simulink model "dft_polyphase_channelizer_32_by_8"  (R2018b)
settings: Solver=FixedStepDiscrete  StartTime=0.0  StopTime=t(end)  RelTol=1e-3  EnableMultiTasking=on
InitFcn:
  | M = 32; % Number of channels in the filter bank.
  | N = 8;  % Number of taps in each FIR filter.
  | n_out = 4000; % Number of output samples
  | datatypeselector = 'hdl'; % 'double' 'single' 'hdl' 'dsp'
  | fidatatype = 'Fixed'; % 'Fixed' 'ScaledDouble'
  | [T,B,U,b,u,t,fs] = generate_inputs(M,N,n_out,datatypeselector,fidatatype);
values from neighbouring files (symbols this model uses):
  B = cast(B,'like',T.fir_filter.coeff)    [generate_inputs.m]    (also in test_real_resource_shared_QR.m = cast(B,'like',A))
  fs = n    [generate_inputs.m]
  T = dft_polyphase_filter_types(datatypeselector,fidatatype,prototypevalue,max(abs(b)))    [generate_inputs.m]
(part 1 of 2)
settings Model: FPTRunName=ScaledDouble  Creator=tbryan  LastModifiedBy=tbryan
settings SolverCC: AutoInsertRateTranBlk=on
settings OptimizationCC: LifeSpan=inf
settings DebuggingCC: ParameterDowncastMsg=none  ParameterOverflowMsg=none  ParameterPrecisionLossMsg=none  ParameterTunabilityLossMsg=none  AllowSymbolicDim=off  LibraryContextMissingDiagnostic=none  SFUnexpectedBacktrackingDiag=warning  SFNoUnconditionalDefaultTransitionDiag=warning  SFExecutionAtInitializationDiag=none
settings HardwareCC: ProdBitPerPointer=32  ProdBitPerSizeT=32  ProdBitPerPtrDiffT=32  ProdLargestAtomicFloat=None  ProdIntDivRoundTo=Undefined  ProdEndianess=Unspecified  ProdWordSize=32  ProdHWDeviceType=ASIC/FPGA->ASIC/FPGA  TargetBitPerLong=64  TargetBitPerPointer=64  TargetBitPerSizeT=64  TargetBitPerPtrDiffT=64  TargetLongLongMode=on  TargetIntDivRoundTo=Zero  TargetEndianess=LittleEndian  TargetWordSize=64  TargetHWDeviceType=MATLAB Host  ProdEqTarget=off
settings SFSimCC: SimUseLocalCustomCode=off
settings RTWCC: RTWUseLocalCustomCode=off
settings CodeAppCC: StateflowObjectComments=on
settings GRTTargetCC: TargetLangStandard=C89/C90 (ANSI)  GeneratePreprocessorConditionals=Disable all
settings ConfigComp: CovMetricSettings=dw  CovHtmlReporting=on  CovSaveCumulativeToWorkspaceVar=on  CovSaveSingleToWorkspaceVar=on  CovExternalEMLEnable=off

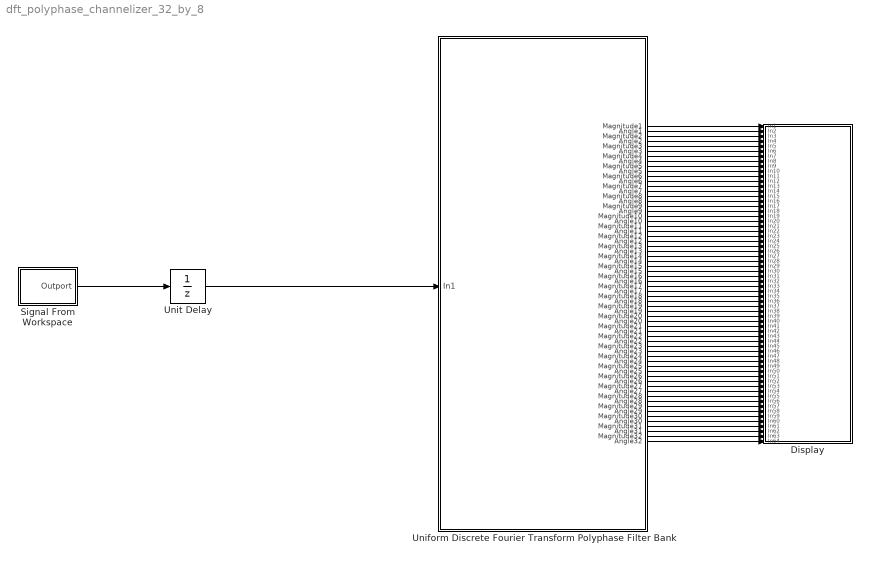
== system dft_polyphase_channelizer_32_by_8 ==
  Display : Subsystem
  Signal From Workspace : Subsystem  mask(Signal From Workspace){X=u, Ts=1/fs, nsamps=1, OutputAfterFinalValue=Setting to zero, ignoreOrWarnInputAndFrameLengths=off, OutputFrames=off}
      mask prompts: X "Signal:"; Ts "Sample time:"; nsamps "Samples per frame:"; OutputAfterFinalValue "Form output after final data value by:"; ignoreOrWarnInputAndFrameLengths "Warn when frame size does not evenly divide input length"; OutputFrames "Output Frames"
      mask help:
      | Output signal samples obtained from the MATLAB workspace at successive sample times.  A signal matrix is interpreted as having one channel per column.  Signal columns may be buffered into frames by specifying a number of samples per frame greater than 1.
      |
      | An M x N x P signal array outputs M x N matrices at successive sample times.  The samples per frame must be equal to 1 for three-dimensional signal arrays.
      mask init:
      | dispX = get_param(gcbh, 'X');
      | [s,Ts] = dspblksfw2('init', X,Ts,nsamps);
      mask Help: eval('blocksethelp');
      mask TypeOptions OutputAfterFinalValue: Setting to zero | Holding final value | Cyclic repetition
      mask Callback OutputAfterFinalValue: dspblksfw2
      mask Display: disp(dispX)
  Uniform Discrete Fourier Transform Polyphase Filter Bank : Subsystem
  Unit Delay : UnitDelay  SampleTime=1/fs
  wires:
  Unit Delay/1 -> Uniform Discrete Fourier Transform Polyphase Filter Bank/1(In1)
  Signal From Workspace/1(Outport) -> Unit Delay/1
  Uniform Discrete Fourier Transform Polyphase Filter Bank/1(Magnitude1) -> Display/1(In1)
  Uniform Discrete Fourier Transform Polyphase Filter Bank/2(Angle1) -> Display/2(In2)
  Uniform Discrete Fourier Transform Polyphase Filter Bank/3(Magnitude2) -> Display/3(In3)
  Uniform Discrete Fourier Transform Polyphase Filter Bank/4(Angle2) -> Display/4(In4)
  Uniform Discrete Fourier Transform Polyphase Filter Bank/5(Magnitude3) -> Display/5(In5)
  Uniform Discrete Fourier Transform Polyphase Filter Bank/6(Angle3) -> Display/6(In6)
  Uniform Discrete Fourier Transform Polyphase Filter Bank/7(Magnitude4) -> Display/7(In7)
  Uniform Discrete Fourier Transform Polyphase Filter Bank/8(Angle4) -> Display/8(In8)
  Uniform Discrete Fourier Transform Polyphase Filter Bank/9(Magnitude5) -> Display/9(In9)
  Uniform Discrete Fourier Transform Polyphase Filter Bank/10(Angle5) -> Display/10(In10)
  Uniform Discrete Fourier Transform Polyphase Filter Bank/11(Magnitude6) -> Display/11(In11)
  Uniform Discrete Fourier Transform Polyphase Filter Bank/12(Angle6) -> Display/12(In12)
  Uniform Discrete Fourier Transform Polyphase Filter Bank/13(Magnitude7) -> Display/13(In13)
  Uniform Discrete Fourier Transform Polyphase Filter Bank/14(Angle7) -> Display/14(In14)
  Uniform Discrete Fourier Transform Polyphase Filter Bank/15(Magnitude8) -> Display/15(In15)
  Uniform Discrete Fourier Transform Polyphase Filter Bank/16(Angle8) -> Display/16(In16)
  Uniform Discrete Fourier Transform Polyphase Filter Bank/17(Magnitude9) -> Display/17(In17)
  Uniform Discrete Fourier Transform Polyphase Filter Bank/18(Angle9) -> Display/18(In18)
  Uniform Discrete Fourier Transform Polyphase Filter Bank/19(Magnitude10) -> Display/19(In19)
  Uniform Discrete Fourier Transform Polyphase Filter Bank/20(Angle10) -> Display/20(In20)
  Uniform Discrete Fourier Transform Polyphase Filter Bank/21(Magnitude11) -> Display/21(In21)
  Uniform Discrete Fourier Transform Polyphase Filter Bank/22(Angle11) -> Display/22(In22)
  Uniform Discrete Fourier Transform Polyphase Filter Bank/23(Magnitude12) -> Display/23(In23)
  Uniform Discrete Fourier Transform Polyphase Filter Bank/24(Angle12) -> Display/24(In24)
  Uniform Discrete Fourier Transform Polyphase Filter Bank/25(Magnitude13) -> Display/25(In25)
  Uniform Discrete Fourier Transform Polyphase Filter Bank/26(Angle13) -> Display/26(In26)
  Uniform Discrete Fourier Transform Polyphase Filter Bank/27(Magnitude14) -> Display/27(In27)
  Uniform Discrete Fourier Transform Polyphase Filter Bank/28(Angle14) -> Display/28(In28)
  Uniform Discrete Fourier Transform Polyphase Filter Bank/29(Magnitude15) -> Display/29(In29)
  Uniform Discrete Fourier Transform Polyphase Filter Bank/30(Angle15) -> Display/30(In30)
  Uniform Discrete Fourier Transform Polyphase Filter Bank/31(Magnitude16) -> Display/31(In31)
  Uniform Discrete Fourier Transform Polyphase Filter Bank/32(Angle16) -> Display/32(In32)
  Uniform Discrete Fourier Transform Polyphase Filter Bank/33(Magnitude17) -> Display/33(In33)
  Uniform Discrete Fourier Transform Polyphase Filter Bank/34(Angle17) -> Display/34(In34)
  Uniform Discrete Fourier Transform Polyphase Filter Bank/35(Magnitude18) -> Display/35(In35)
  Uniform Discrete Fourier Transform Polyphase Filter Bank/36(Angle18) -> Display/36(In36)
  Uniform Discrete Fourier Transform Polyphase Filter Bank/37(Magnitude19) -> Display/37(In37)
  Uniform Discrete Fourier Transform Polyphase Filter Bank/38(Angle19) -> Display/38(In38)
  Uniform Discrete Fourier Transform Polyphase Filter Bank/39(Magnitude20) -> Display/39(In39)
  Uniform Discrete Fourier Transform Polyphase Filter Bank/40(Angle20) -> Display/40(In40)
  Uniform Discrete Fourier Transform Polyphase Filter Bank/41(Magnitude21) -> Display/41(In41)
  Uniform Discrete Fourier Transform Polyphase Filter Bank/42(Angle21) -> Display/42(In42)
  Uniform Discrete Fourier Transform Polyphase Filter Bank/43(Magnitude22) -> Display/43(In43)
  Uniform Discrete Fourier Transform Polyphase Filter Bank/44(Angle22) -> Display/44(In44)
  Uniform Discrete Fourier Transform Polyphase Filter Bank/45(Magnitude23) -> Display/45(In45)
  Uniform Discrete Fourier Transform Polyphase Filter Bank/46(Angle23) -> Display/46(In46)
  Uniform Discrete Fourier Transform Polyphase Filter Bank/47(Magnitude24) -> Display/47(In47)
  Uniform Discrete Fourier Transform Polyphase Filter Bank/48(Angle24) -> Display/48(In48)
  Uniform Discrete Fourier Transform Polyphase Filter Bank/49(Magnitude25) -> Display/49(In49)
  Uniform Discrete Fourier Transform Polyphase Filter Bank/50(Angle25) -> Display/50(In50)
  Uniform Discrete Fourier Transform Polyphase Filter Bank/51(Magnitude26) -> Display/51(In51)
  Uniform Discrete Fourier Transform Polyphase Filter Bank/52(Angle26) -> Display/52(In52)
  Uniform Discrete Fourier Transform Polyphase Filter Bank/53(Magnitude27) -> Display/53(In53)
  Uniform Discrete Fourier Transform Polyphase Filter Bank/54(Angle27) -> Display/54(In54)
  Uniform Discrete Fourier Transform Polyphase Filter Bank/55(Magnitude28) -> Display/55(In55)
  Uniform Discrete Fourier Transform Polyphase Filter Bank/56(Angle28) -> Display/56(In56)
  Uniform Discrete Fourier Transform Polyphase Filter Bank/57(Magnitude29) -> Display/57(In57)
  Uniform Discrete Fourier Transform Polyphase Filter Bank/58(Angle29) -> Display/58(In58)
  Uniform Discrete Fourier Transform Polyphase Filter Bank/59(Magnitude30) -> Display/59(In59)
  Uniform Discrete Fourier Transform Polyphase Filter Bank/60(Angle30) -> Display/60(In60)
  Uniform Discrete Fourier Transform Polyphase Filter Bank/61(Magnitude31) -> Display/61(In61)
  Uniform Discrete Fourier Transform Polyphase Filter Bank/62(Angle31) -> Display/62(In62)
  Uniform Discrete Fourier Transform Polyphase Filter Bank/63(Magnitude32) -> Display/63(In63)
  Uniform Discrete Fourier Transform Polyphase Filter Bank/64(Angle32) -> Display/64(In64)

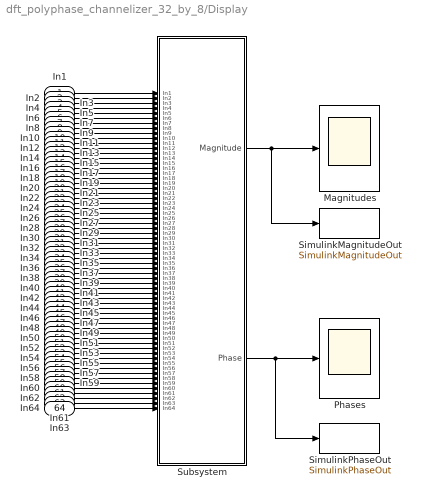
== system dft_polyphase_channelizer_32_by_8/Display ==
  In1 : Inport
  In2 : Inport  Port=2
  In3 : Inport  Port=3
  In4 : Inport  Port=4
  In5 : Inport  Port=5
  In6 : Inport  Port=6
  In7 : Inport  Port=7
  In8 : Inport  Port=8
  In9 : Inport  Port=9
  In10 : Inport  Port=10
  In11 : Inport  Port=11
  In12 : Inport  Port=12
  In13 : Inport  Port=13
  In14 : Inport  Port=14
  In15 : Inport  Port=15
  In16 : Inport  Port=16
  In17 : Inport  Port=17
  In18 : Inport  Port=18
  In19 : Inport  Port=19
  In20 : Inport  Port=20
  In21 : Inport  Port=21
  In22 : Inport  Port=22
  In23 : Inport  Port=23
  In24 : Inport  Port=24
  In25 : Inport  Port=25
  In26 : Inport  Port=26
  In27 : Inport  Port=27
  In28 : Inport  Port=28
  In29 : Inport  Port=29
  In30 : Inport  Port=30
  In31 : Inport  Port=31
  In32 : Inport  Port=32
  In33 : Inport  Port=33
  In34 : Inport  Port=34
  In35 : Inport  Port=35
  In36 : Inport  Port=36
  In37 : Inport  Port=37
  In38 : Inport  Port=38
  In39 : Inport  Port=39
  In40 : Inport  Port=40
  In41 : Inport  Port=41
  In42 : Inport  Port=42
  In43 : Inport  Port=43
  In44 : Inport  Port=44
  In45 : Inport  Port=45
  In46 : Inport  Port=46
  In47 : Inport  Port=47
  In48 : Inport  Port=48
  In49 : Inport  Port=49
  In50 : Inport  Port=50
  In51 : Inport  Port=51
  In52 : Inport  Port=52
  In53 : Inport  Port=53
  In54 : Inport  Port=54
  In55 : Inport  Port=55
  In56 : Inport  Port=56
  In57 : Inport  Port=57
  In58 : Inport  Port=58
  In59 : Inport  Port=59
  In60 : Inport  Port=60
  In61 : Inport  Port=61
  In62 : Inport  Port=62
  In63 : Inport  Port=63
  In64 : Inport  Port=64
  Magnitudes : Scope
  Phases : Scope
  SimulinkMagnitudeOut : ToWorkspace  VariableName=SimulinkMagnitudeOut  SampleTime=-1
      settings: Save2DSignal=2-D array (concatenate along first dimension)
  SimulinkPhaseOut : ToWorkspace  VariableName=SimulinkPhaseOut  SampleTime=-1
      settings: Save2DSignal=2-D array (concatenate along first dimension)
  Subsystem : Subsystem
  wires:
  In8/1 -> Subsystem/8(In8)
  In43/1 -> Subsystem/43(In43)
  In21/1 -> Subsystem/21(In21)
  In35/1 -> Subsystem/35(In35)
  In33/1 -> Subsystem/33(In33)
  In26/1 -> Subsystem/26(In26)
  In30/1 -> Subsystem/30(In30)
  In27/1 -> Subsystem/27(In27)
  In23/1 -> Subsystem/23(In23)
  In20/1 -> Subsystem/20(In20)
  In5/1 -> Subsystem/5(In5)
  In63/1 -> Subsystem/63(In63)
  In10/1 -> Subsystem/10(In10)
  In61/1 -> Subsystem/61(In61)
  In41/1 -> Subsystem/41(In41)
  In6/1 -> Subsystem/6(In6)
  In49/1 -> Subsystem/49(In49)
  In53/1 -> Subsystem/53(In53)
  In47/1 -> Subsystem/47(In47)
  In55/1 -> Subsystem/55(In55)
  In13/1 -> Subsystem/13(In13)
  In32/1 -> Subsystem/32(In32)
  In14/1 -> Subsystem/14(In14)
  In38/1 -> Subsystem/38(In38)
  In17/1 -> Subsystem/17(In17)
  In1/1 -> Subsystem/1(In1)
  In62/1 -> Subsystem/62(In62)
  In46/1 -> Subsystem/46(In46)
  In44/1 -> Subsystem/44(In44)
  In58/1 -> Subsystem/58(In58)
  In12/1 -> Subsystem/12(In12)
  In19/1 -> Subsystem/19(In19)
  In15/1 -> Subsystem/15(In15)
  In16/1 -> Subsystem/16(In16)
  In18/1 -> Subsystem/18(In18)
  In24/1 -> Subsystem/24(In24)
  In29/1 -> Subsystem/29(In29)
  In2/1 -> Subsystem/2(In2)
  In3/1 -> Subsystem/3(In3)
  In7/1 -> Subsystem/7(In7)
  In4/1 -> Subsystem/4(In4)
  In28/1 -> Subsystem/28(In28)
  In9/1 -> Subsystem/9(In9)
  In22/1 -> Subsystem/22(In22)
  Subsystem/2(Phase) -> SimulinkPhaseOut/1, Phases/1
  In57/1 -> Subsystem/57(In57)
  In36/1 -> Subsystem/36(In36)
  In50/1 -> Subsystem/50(In50)
  In34/1 -> Subsystem/34(In34)
  In56/1 -> Subsystem/56(In56)
  In11/1 -> Subsystem/11(In11)
  In64/1 -> Subsystem/64(In64)
  Subsystem/1(Magnitude) -> SimulinkMagnitudeOut/1, Magnitudes/1
  In25/1 -> Subsystem/25(In25)
  In59/1 -> Subsystem/59(In59)
  In39/1 -> Subsystem/39(In39)
  In45/1 -> Subsystem/45(In45)
  In42/1 -> Subsystem/42(In42)
  In52/1 -> Subsystem/52(In52)
  In60/1 -> Subsystem/60(In60)
  In48/1 -> Subsystem/48(In48)
  In51/1 -> Subsystem/51(In51)
  In54/1 -> Subsystem/54(In54)
  In31/1 -> Subsystem/31(In31)
  In37/1 -> Subsystem/37(In37)
  In40/1 -> Subsystem/40(In40)

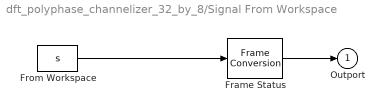
== system dft_polyphase_channelizer_32_by_8/Signal From Workspace ==
  Frame Status : FrameConversion  OutFrame=Sample-based
  From Workspace : FromWorkspace  VariableName=s  SampleTime=Ts  Interpolate=off  OutputAfterFinalValue=Setting to zero
  Outport : Outport  InitialOutput=0
  wires:
  Frame Status/1 -> Outport/1
  From Workspace/1 -> Frame Status/1

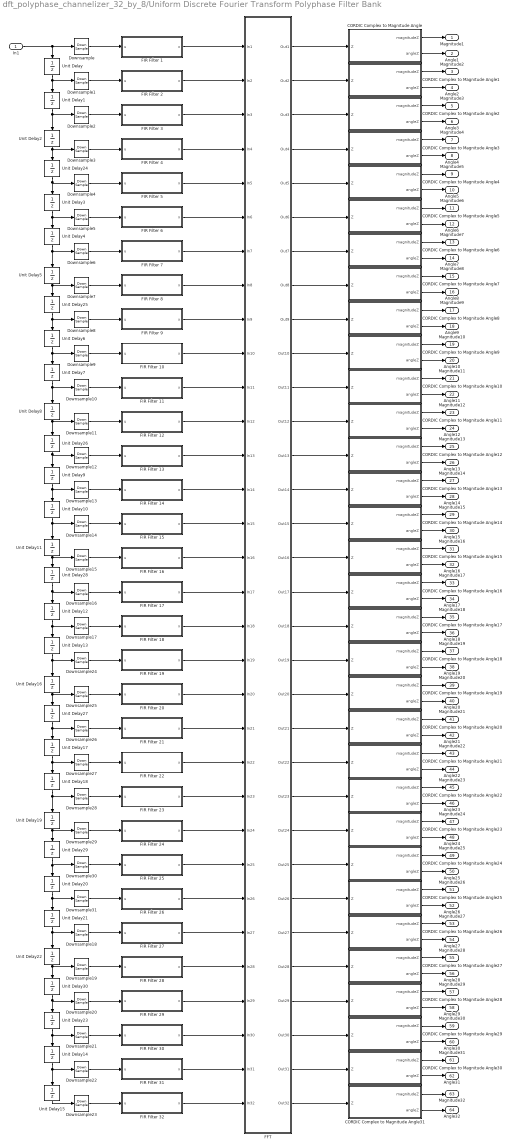
== system dft_polyphase_channelizer_32_by_8/Uniform Discrete Fourier Transform Polyphase Filter Bank ==
  In1 : Inport
  " CORDIC Complex to Magnitude Angle" : MATLAB Function  TreatAsAtomicUnit=on
  " CORDIC Complex to Magnitude Angle1" : MATLAB Function  TreatAsAtomicUnit=on
  " CORDIC Complex to Magnitude Angle10" : MATLAB Function  TreatAsAtomicUnit=on
  " CORDIC Complex to Magnitude Angle11" : MATLAB Function  TreatAsAtomicUnit=on
  " CORDIC Complex to Magnitude Angle12" : MATLAB Function  TreatAsAtomicUnit=on
  " CORDIC Complex to Magnitude Angle13" : MATLAB Function  TreatAsAtomicUnit=on
  " CORDIC Complex to Magnitude Angle14" : MATLAB Function  TreatAsAtomicUnit=on
  " CORDIC Complex to Magnitude Angle15" : MATLAB Function  TreatAsAtomicUnit=on
  " CORDIC Complex to Magnitude Angle16" : MATLAB Function  TreatAsAtomicUnit=on
  " CORDIC Complex to Magnitude Angle17" : MATLAB Function  TreatAsAtomicUnit=on
  " CORDIC Complex to Magnitude Angle18" : MATLAB Function  TreatAsAtomicUnit=on
  " CORDIC Complex to Magnitude Angle19" : MATLAB Function  TreatAsAtomicUnit=on
  " CORDIC Complex to Magnitude Angle2" : MATLAB Function  TreatAsAtomicUnit=on
  " CORDIC Complex to Magnitude Angle20" : MATLAB Function  TreatAsAtomicUnit=on
  " CORDIC Complex to Magnitude Angle21" : MATLAB Function  TreatAsAtomicUnit=on
  " CORDIC Complex to Magnitude Angle22" : MATLAB Function  TreatAsAtomicUnit=on
  " CORDIC Complex to Magnitude Angle23" : MATLAB Function  TreatAsAtomicUnit=on
  " CORDIC Complex to Magnitude Angle24" : MATLAB Function  TreatAsAtomicUnit=on
  " CORDIC Complex to Magnitude Angle25" : MATLAB Function  TreatAsAtomicUnit=on
  " CORDIC Complex to Magnitude Angle26" : MATLAB Function  TreatAsAtomicUnit=on
  " CORDIC Complex to Magnitude Angle27" : MATLAB Function  TreatAsAtomicUnit=on
  " CORDIC Complex to Magnitude Angle28" : MATLAB Function  TreatAsAtomicUnit=on
  " CORDIC Complex to Magnitude Angle29" : MATLAB Function  TreatAsAtomicUnit=on
  " CORDIC Complex to Magnitude Angle3" : MATLAB Function  TreatAsAtomicUnit=on
  " CORDIC Complex to Magnitude Angle30" : MATLAB Function  TreatAsAtomicUnit=on
  " CORDIC Complex to Magnitude Angle31" : MATLAB Function  TreatAsAtomicUnit=on
  " CORDIC Complex to Magnitude Angle4" : MATLAB Function  TreatAsAtomicUnit=on
  " CORDIC Complex to Magnitude Angle5" : MATLAB Function  TreatAsAtomicUnit=on
  " CORDIC Complex to Magnitude Angle6" : MATLAB Function  TreatAsAtomicUnit=on
  " CORDIC Complex to Magnitude Angle7" : MATLAB Function  TreatAsAtomicUnit=on
  " CORDIC Complex to Magnitude Angle8" : MATLAB Function  TreatAsAtomicUnit=on
  " CORDIC Complex to Magnitude Angle9" : MATLAB Function  TreatAsAtomicUnit=on
  Downsample{,1..31} (32 alike) : DownSample  N=M  RateOptions=Allow multirate processing
  FFT : Subsystem
      mask Display: disp('FFT')
  FIR Filter 1 : MATLAB Function  TreatAsAtomicUnit=on  mask{b=B(1,:), T=T.fir_filter}
      mask prompts: b "Coefficients: b from MATLAB's filter(b,1,x)"
  FIR Filter 10 : MATLAB Function  TreatAsAtomicUnit=on  mask{b=B(10,:), T=T.fir_filter}
      mask prompts: b "Coefficients: b from MATLAB's filter(b,1,x)"
  FIR Filter 11 : MATLAB Function  TreatAsAtomicUnit=on  mask{b=B(11,:), T=T.fir_filter}
      mask prompts: b "Coefficients: b from MATLAB's filter(b,1,x)"
  FIR Filter 12 : MATLAB Function  TreatAsAtomicUnit=on  mask{b=B(12,:), T=T.fir_filter}
      mask prompts: b "Coefficients: b from MATLAB's filter(b,1,x)"
  FIR Filter 13 : MATLAB Function  TreatAsAtomicUnit=on  mask{b=B(13,:), T=T.fir_filter}
      mask prompts: b "Coefficients: b from MATLAB's filter(b,1,x)"
  FIR Filter 14 : MATLAB Function  TreatAsAtomicUnit=on  mask{b=B(14,:), T=T.fir_filter}
      mask prompts: b "Coefficients: b from MATLAB's filter(b,1,x)"
  FIR Filter 15 : MATLAB Function  TreatAsAtomicUnit=on  mask{b=B(15,:), T=T.fir_filter}
      mask prompts: b "Coefficients: b from MATLAB's filter(b,1,x)"
  FIR Filter 16 : MATLAB Function  TreatAsAtomicUnit=on  mask{b=B(16,:), T=T.fir_filter}
      mask prompts: b "Coefficients: b from MATLAB's filter(b,1,x)"
  FIR Filter 17 : MATLAB Function  TreatAsAtomicUnit=on  mask{b=B(17,:), T=T.fir_filter}
      mask prompts: b "Coefficients: b from MATLAB's filter(b,1,x)"
  FIR Filter 18 : MATLAB Function  TreatAsAtomicUnit=on  mask{b=B(18,:), T=T.fir_filter}
      mask prompts: b "Coefficients: b from MATLAB's filter(b,1,x)"
  FIR Filter 19 : MATLAB Function  TreatAsAtomicUnit=on  mask{b=B(19,:), T=T.fir_filter}
      mask prompts: b "Coefficients: b from MATLAB's filter(b,1,x)"
  FIR Filter 2 : MATLAB Function  TreatAsAtomicUnit=on  mask{b=B(2,:), T=T.fir_filter}
      mask prompts: b "Coefficients: b from MATLAB's filter(b,1,x)"
  FIR Filter 20 : MATLAB Function  TreatAsAtomicUnit=on  mask{b=B(20,:), T=T.fir_filter}
      mask prompts: b "Coefficients: b from MATLAB's filter(b,1,x)"
  FIR Filter 21 : MATLAB Function  TreatAsAtomicUnit=on  mask{b=B(21,:), T=T.fir_filter}
      mask prompts: b "Coefficients: b from MATLAB's filter(b,1,x)"
  FIR Filter 22 : MATLAB Function  TreatAsAtomicUnit=on  mask{b=B(22,:), T=T.fir_filter}
      mask prompts: b "Coefficients: b from MATLAB's filter(b,1,x)"
  FIR Filter 23 : MATLAB Function  TreatAsAtomicUnit=on  mask{b=B(23,:), T=T.fir_filter}
      mask prompts: b "Coefficients: b from MATLAB's filter(b,1,x)"
  FIR Filter 24 : MATLAB Function  TreatAsAtomicUnit=on  mask{b=B(24,:), T=T.fir_filter}
      mask prompts: b "Coefficients: b from MATLAB's filter(b,1,x)"
  FIR Filter 25 : MATLAB Function  TreatAsAtomicUnit=on  mask{b=B(25,:), T=T.fir_filter}
      mask prompts: b "Coefficients: b from MATLAB's filter(b,1,x)"
  FIR Filter 26 : MATLAB Function  TreatAsAtomicUnit=on  mask{b=B(26,:), T=T.fir_filter}
      mask prompts: b "Coefficients: b from MATLAB's filter(b,1,x)"
  FIR Filter 27 : MATLAB Function  TreatAsAtomicUnit=on  mask{b=B(27,:), T=T.fir_filter}
      mask prompts: b "Coefficients: b from MATLAB's filter(b,1,x)"
  FIR Filter 28 : MATLAB Function  TreatAsAtomicUnit=on  mask{b=B(28,:), T=T.fir_filter}
      mask prompts: b "Coefficients: b from MATLAB's filter(b,1,x)"
  FIR Filter 29 : MATLAB Function  TreatAsAtomicUnit=on  mask{b=B(29,:), T=T.fir_filter}
      mask prompts: b "Coefficients: b from MATLAB's filter(b,1,x)"
  FIR Filter 3 : MATLAB Function  TreatAsAtomicUnit=on  mask{b=B(3,:), T=T.fir_filter}
      mask prompts: b "Coefficients: b from MATLAB's filter(b,1,x)"
  FIR Filter 30 : MATLAB Function  TreatAsAtomicUnit=on  mask{b=B(30,:), T=T.fir_filter}
      mask prompts: b "Coefficients: b from MATLAB's filter(b,1,x)"
  FIR Filter 31 : MATLAB Function  TreatAsAtomicUnit=on  mask{b=B(31,:), T=T.fir_filter}
      mask prompts: b "Coefficients: b from MATLAB's filter(b,1,x)"
  FIR Filter 32 : MATLAB Function  TreatAsAtomicUnit=on  mask{b=B(32,:), T=T.fir_filter}
      mask prompts: b "Coefficients: b from MATLAB's filter(b,1,x)"
  FIR Filter 4 : MATLAB Function  TreatAsAtomicUnit=on  mask{b=B(4,:), T=T.fir_filter}
      mask prompts: b "Coefficients: b from MATLAB's filter(b,1,x)"
  FIR Filter 5 : MATLAB Function  TreatAsAtomicUnit=on  mask{b=B(5,:), T=T.fir_filter}
      mask prompts: b "Coefficients: b from MATLAB's filter(b,1,x)"
  FIR Filter 6 : MATLAB Function  TreatAsAtomicUnit=on  mask{b=B(6,:), T=T.fir_filter}
      mask prompts: b "Coefficients: b from MATLAB's filter(b,1,x)"
  FIR Filter 7 : MATLAB Function  TreatAsAtomicUnit=on  mask{b=B(7,:), T=T.fir_filter}
      mask prompts: b "Coefficients: b from MATLAB's filter(b,1,x)"
  FIR Filter 8 : MATLAB Function  TreatAsAtomicUnit=on  mask{b=B(8,:), T=T.fir_filter}
      mask prompts: b "Coefficients: b from MATLAB's filter(b,1,x)"
  FIR Filter 9 : MATLAB Function  TreatAsAtomicUnit=on  mask{b=B(9,:), T=T.fir_filter}
      mask prompts: b "Coefficients: b from MATLAB's filter(b,1,x)"
  Unit Delay{,1..30} (31 alike) : UnitDelay  SampleTime=-1
  Magnitude1 : Outport
  Angle1 : Outport  Port=2
  Magnitude2 : Outport  Port=3
  Angle2 : Outport  Port=4
  Magnitude3 : Outport  Port=5
  Angle3 : Outport  Port=6
  Magnitude4 : Outport  Port=7
  Angle4 : Outport  Port=8
  Magnitude5 : Outport  Port=9
  Angle5 : Outport  Port=10
  Magnitude6 : Outport  Port=11
  Angle6 : Outport  Port=12
  Magnitude7 : Outport  Port=13
  Angle7 : Outport  Port=14
  Magnitude8 : Outport  Port=15
  Angle8 : Outport  Port=16
  Magnitude9 : Outport  Port=17
  Angle9 : Outport  Port=18
  Magnitude10 : Outport  Port=19
  Angle10 : Outport  Port=20
  Magnitude11 : Outport  Port=21
  Angle11 : Outport  Port=22
  Magnitude12 : Outport  Port=23
  Angle12 : Outport  Port=24
  Magnitude13 : Outport  Port=25
  Angle13 : Outport  Port=26
  Magnitude14 : Outport  Port=27
  Angle14 : Outport  Port=28
  Magnitude15 : Outport  Port=29
  Angle15 : Outport  Port=30
  Magnitude16 : Outport  Port=31
  Angle16 : Outport  Port=32
  Magnitude17 : Outport  Port=33
  Angle17 : Outport  Port=34
  Magnitude18 : Outport  Port=35
  Angle18 : Outport  Port=36
  Magnitude19 : Outport  Port=37
  Angle19 : Outport  Port=38
  Magnitude20 : Outport  Port=39
  Angle20 : Outport  Port=40
  Magnitude21 : Outport  Port=41
  Angle21 : Outport  Port=42
  Magnitude22 : Outport  Port=43
  Angle22 : Outport  Port=44
  Magnitude23 : Outport  Port=45
  Angle23 : Outport  Port=46
  Magnitude24 : Outport  Port=47
  Angle24 : Outport  Port=48
  Magnitude25 : Outport  Port=49
  Angle25 : Outport  Port=50
  Magnitude26 : Outport  Port=51
  Angle26 : Outport  Port=52
  Magnitude27 : Outport  Port=53
  Angle27 : Outport  Port=54
  Magnitude28 : Outport  Port=55
  Angle28 : Outport  Port=56
  Magnitude29 : Outport  Port=57
  Angle29 : Outport  Port=58
  Magnitude30 : Outport  Port=59
  Angle30 : Outport  Port=60
  Magnitude31 : Outport  Port=61
  Angle31 : Outport  Port=62
  Magnitude32 : Outport  Port=63
  Angle32 : Outport  Port=64
  wires:
  " CORDIC Complex to Magnitude Angle1"/2(angleZ) -> Angle2/1
  " CORDIC Complex to Magnitude Angle"/1(magnitudeZ) -> Magnitude1/1
  " CORDIC Complex to Magnitude Angle2"/2(angleZ) -> Angle3/1
  " CORDIC Complex to Magnitude Angle3"/2(angleZ) -> Angle4/1
  " CORDIC Complex to Magnitude Angle2"/1(magnitudeZ) -> Magnitude3/1
  " CORDIC Complex to Magnitude Angle"/2(angleZ) -> Angle1/1
  " CORDIC Complex to Magnitude Angle3"/1(magnitudeZ) -> Magnitude4/1
  Downsample/1 -> FIR Filter 1/1(u)
  Unit Delay/1 -> Unit Delay1/1, Downsample1/1
  Unit Delay1/1 -> Unit Delay2/1, Downsample2/1
  Unit Delay2/1 -> Unit Delay24/1, Downsample3/1
  " CORDIC Complex to Magnitude Angle1"/1(magnitudeZ) -> Magnitude2/1
  Unit Delay3/1 -> Unit Delay4/1, Downsample5/1
  Unit Delay4/1 -> Unit Delay5/1, Downsample6/1
  Unit Delay6/1 -> Unit Delay7/1, Downsample9/1
  Unit Delay7/1 -> Unit Delay8/1, Downsample10/1
  Unit Delay8/1 -> Unit Delay26/1, Downsample11/1
  Unit Delay9/1 -> Unit Delay10/1, Downsample13/1
  Unit Delay10/1 -> Unit Delay11/1, Downsample14/1
  Unit Delay11/1 -> Unit Delay28/1, Downsample15/1
  Unit Delay12/1 -> Unit Delay13/1, Downsample17/1
  Unit Delay13/1 -> Unit Delay16/1, Downsample24/1
  Unit Delay16/1 -> Unit Delay27/1, Downsample25/1
  Unit Delay17/1 -> Unit Delay18/1, Downsample27/1
  Unit Delay18/1 -> Unit Delay19/1, Downsample28/1
  Unit Delay19/1 -> Unit Delay29/1, Downsample29/1
  Unit Delay20/1 -> Unit Delay21/1, Downsample31/1
  Unit Delay21/1 -> Unit Delay22/1, Downsample18/1
  Unit Delay22/1 -> Unit Delay30/1, Downsample19/1
  Unit Delay23/1 -> Unit Delay14/1, Downsample21/1
  Unit Delay14/1 -> Unit Delay15/1, Downsample22/1
  Unit Delay15/1 -> Downsample23/1
  " CORDIC Complex to Magnitude Angle5"/2(angleZ) -> Angle6/1
  " CORDIC Complex to Magnitude Angle4"/1(magnitudeZ) -> Magnitude5/1
  " CORDIC Complex to Magnitude Angle6"/2(angleZ) -> Angle7/1
  " CORDIC Complex to Magnitude Angle7"/2(angleZ) -> Angle8/1
  " CORDIC Complex to Magnitude Angle6"/1(magnitudeZ) -> Magnitude7/1
  " CORDIC Complex to Magnitude Angle4"/2(angleZ) -> Angle5/1
  " CORDIC Complex to Magnitude Angle7"/1(magnitudeZ) -> Magnitude8/1
  " CORDIC Complex to Magnitude Angle5"/1(magnitudeZ) -> Magnitude6/1
  " CORDIC Complex to Magnitude Angle9"/2(angleZ) -> Angle10/1
  " CORDIC Complex to Magnitude Angle8"/1(magnitudeZ) -> Magnitude9/1
  " CORDIC Complex to Magnitude Angle10"/2(angleZ) -> Angle11/1
  " CORDIC Complex to Magnitude Angle11"/2(angleZ) -> Angle12/1
  " CORDIC Complex to Magnitude Angle10"/1(magnitudeZ) -> Magnitude11/1
  " CORDIC Complex to Magnitude Angle8"/2(angleZ) -> Angle9/1
  " CORDIC Complex to Magnitude Angle11"/1(magnitudeZ) -> Magnitude12/1
  " CORDIC Complex to Magnitude Angle9"/1(magnitudeZ) -> Magnitude10/1
  " CORDIC Complex to Magnitude Angle13"/2(angleZ) -> Angle14/1
  " CORDIC Complex to Magnitude Angle12"/1(magnitudeZ) -> Magnitude13/1
  " CORDIC Complex to Magnitude Angle14"/2(angleZ) -> Angle15/1
  " CORDIC Complex to Magnitude Angle15"/2(angleZ) -> Angle16/1
  " CORDIC Complex to Magnitude Angle14"/1(magnitudeZ) -> Magnitude15/1
  " CORDIC Complex to Magnitude Angle12"/2(angleZ) -> Angle13/1
  " CORDIC Complex to Magnitude Angle15"/1(magnitudeZ) -> Magnitude16/1
  " CORDIC Complex to Magnitude Angle13"/1(magnitudeZ) -> Magnitude14/1
  " CORDIC Complex to Magnitude Angle17"/2(angleZ) -> Angle18/1
  " CORDIC Complex to Magnitude Angle16"/1(magnitudeZ) -> Magnitude17/1
  " CORDIC Complex to Magnitude Angle18"/2(angleZ) -> Angle19/1
  " CORDIC Complex to Magnitude Angle19"/2(angleZ) -> Angle20/1
  " CORDIC Complex to Magnitude Angle18"/1(magnitudeZ) -> Magnitude19/1
  " CORDIC Complex to Magnitude Angle16"/2(angleZ) -> Angle17/1
  " CORDIC Complex to Magnitude Angle19"/1(magnitudeZ) -> Magnitude20/1
  " CORDIC Complex to Magnitude Angle17"/1(magnitudeZ) -> Magnitude18/1
  " CORDIC Complex to Magnitude Angle21"/2(angleZ) -> Angle22/1
  " CORDIC Complex to Magnitude Angle20"/1(magnitudeZ) -> Magnitude21/1
  " CORDIC Complex to Magnitude Angle22"/2(angleZ) -> Angle23/1
  " CORDIC Complex to Magnitude Angle23"/2(angleZ) -> Angle24/1
  " CORDIC Complex to Magnitude Angle22"/1(magnitudeZ) -> Magnitude23/1
  " CORDIC Complex to Magnitude Angle20"/2(angleZ) -> Angle21/1
  " CORDIC Complex to Magnitude Angle23"/1(magnitudeZ) -> Magnitude24/1
  " CORDIC Complex to Magnitude Angle21"/1(magnitudeZ) -> Magnitude22/1
  " CORDIC Complex to Magnitude Angle25"/2(angleZ) -> Angle26/1
  " CORDIC Complex to Magnitude Angle24"/1(magnitudeZ) -> Magnitude25/1
  " CORDIC Complex to Magnitude Angle26"/2(angleZ) -> Angle27/1
  " CORDIC Complex to Magnitude Angle27"/2(angleZ) -> Angle28/1
  " CORDIC Complex to Magnitude Angle26"/1(magnitudeZ) -> Magnitude27/1
  " CORDIC Complex to Magnitude Angle24"/2(angleZ) -> Angle25/1
  " CORDIC Complex to Magnitude Angle27"/1(magnitudeZ) -> Magnitude28/1
  " CORDIC Complex to Magnitude Angle25"/1(magnitudeZ) -> Magnitude26/1
  " CORDIC Complex to Magnitude Angle29"/2(angleZ) -> Angle30/1
  " CORDIC Complex to Magnitude Angle28"/1(magnitudeZ) -> Magnitude29/1
  " CORDIC Complex to Magnitude Angle30"/2(angleZ) -> Angle31/1
  " CORDIC Complex to Magnitude Angle31"/2(angleZ) -> Angle32/1
  " CORDIC Complex to Magnitude Angle30"/1(magnitudeZ) -> Magnitude31/1
  " CORDIC Complex to Magnitude Angle28"/2(angleZ) -> Angle29/1
  " CORDIC Complex to Magnitude Angle31"/1(magnitudeZ) -> Magnitude32/1
  " CORDIC Complex to Magnitude Angle29"/1(magnitudeZ) -> Magnitude30/1
  In1/1 -> Unit Delay/1, Downsample/1
  FIR Filter 1/1(x) -> FFT/1(In1)
  FFT/1(Out1) -> " CORDIC Complex to Magnitude Angle"/1(Z)
  FFT/2(Out2) -> " CORDIC Complex to Magnitude Angle1"/1(Z)
  FFT/3(Out3) -> " CORDIC Complex to Magnitude Angle2"/1(Z)
  FFT/4(Out4) -> " CORDIC Complex to Magnitude Angle3"/1(Z)
  FFT/5(Out5) -> " CORDIC Complex to Magnitude Angle4"/1(Z)
  FFT/6(Out6) -> " CORDIC Complex to Magnitude Angle5"/1(Z)
  FFT/7(Out7) -> " CORDIC Complex to Magnitude Angle6"/1(Z)
  FFT/8(Out8) -> " CORDIC Complex to Magnitude Angle7"/1(Z)
  FFT/9(Out9) -> " CORDIC Complex to Magnitude Angle8"/1(Z)
  FFT/10(Out10) -> " CORDIC Complex to Magnitude Angle9"/1(Z)
  FFT/11(Out11) -> " CORDIC Complex to Magnitude Angle10"/1(Z)
  FFT/12(Out12) -> " CORDIC Complex to Magnitude Angle11"/1(Z)
  FFT/13(Out13) -> " CORDIC Complex to Magnitude Angle12"/1(Z)
  FFT/14(Out14) -> " CORDIC Complex to Magnitude Angle13"/1(Z)
  FFT/15(Out15) -> " CORDIC Complex to Magnitude Angle14"/1(Z)
  FFT/16(Out16) -> " CORDIC Complex to Magnitude Angle15"/1(Z)
  FFT/17(Out17) -> " CORDIC Complex to Magnitude Angle16"/1(Z)
  FFT/18(Out18) -> " CORDIC Complex to Magnitude Angle17"/1(Z)
  FFT/19(Out19) -> " CORDIC Complex to Magnitude Angle18"/1(Z)
  FFT/20(Out20) -> " CORDIC Complex to Magnitude Angle19"/1(Z)
  FFT/21(Out21) -> " CORDIC Complex to Magnitude Angle20"/1(Z)
  FFT/22(Out22) -> " CORDIC Complex to Magnitude Angle21"/1(Z)
  FFT/23(Out23) -> " CORDIC Complex to Magnitude Angle22"/1(Z)
  FFT/24(Out24) -> " CORDIC Complex to Magnitude Angle23"/1(Z)
  FFT/25(Out25) -> " CORDIC Complex to Magnitude Angle24"/1(Z)
  FFT/26(Out26) -> " CORDIC Complex to Magnitude Angle25"/1(Z)
  FFT/30(Out30) -> " CORDIC Complex to Magnitude Angle29"/1(Z)
  FFT/31(Out31) -> " CORDIC Complex to Magnitude Angle30"/1(Z)
  FFT/32(Out32) -> " CORDIC Complex to Magnitude Angle31"/1(Z)
  Unit Delay24/1 -> Downsample4/1, Unit Delay3/1
  Unit Delay25/1 -> Downsample8/1, Unit Delay6/1
  Unit Delay5/1 -> Unit Delay25/1, Downsample7/1
  Unit Delay26/1 -> Downsample12/1, Unit Delay9/1
  Unit Delay27/1 -> Downsample26/1, Unit Delay17/1
  Unit Delay28/1 -> Downsample16/1, Unit Delay12/1
  Unit Delay29/1 -> Downsample30/1, Unit Delay20/1
  Unit Delay30/1 -> Downsample20/1, Unit Delay23/1
  Downsample1/1 -> FIR Filter 2/1(u)
  FIR Filter 2/1(x) -> FFT/2(In2)
  Downsample3/1 -> FIR Filter 4/1(u)
  FIR Filter 4/1(x) -> FFT/4(In4)
  Downsample2/1 -> FIR Filter 3/1(u)
  FIR Filter 3/1(x) -> FFT/3(In3)
  Downsample4/1 -> FIR Filter 5/1(u)
  FIR Filter 5/1(x) -> FFT/5(In5)
  Downsample5/1 -> FIR Filter 6/1(u)
  FIR Filter 6/1(x) -> FFT/6(In6)
  Downsample6/1 -> FIR Filter 7/1(u)
  FIR Filter 7/1(x) -> FFT/7(In7)
  Downsample7/1 -> FIR Filter 8/1(u)
  FIR Filter 8/1(x) -> FFT/8(In8)
  Downsample8/1 -> FIR Filter 9/1(u)
  FIR Filter 9/1(x) -> FFT/9(In9)
  Downsample9/1 -> FIR Filter 10/1(u)
  FIR Filter 10/1(x) -> FFT/10(In10)
  Downsample12/1 -> FIR Filter 13/1(u)
  Downsample11/1 -> FIR Filter 12/1(u)
  Downsample10/1 -> FIR Filter 11/1(u)
  Downsample13/1 -> FIR Filter 14/1(u)
  Downsample14/1 -> FIR Filter 15/1(u)
  Downsample15/1 -> FIR Filter 16/1(u)
  Downsample16/1 -> FIR Filter 17/1(u)
  Downsample17/1 -> FIR Filter 18/1(u)
  Downsample24/1 -> FIR Filter 19/1(u)
  Downsample25/1 -> FIR Filter 20/1(u)
  Downsample26/1 -> FIR Filter 21/1(u)
  Downsample27/1 -> FIR Filter 22/1(u)
  Downsample28/1 -> FIR Filter 23/1(u)
  Downsample29/1 -> FIR Filter 24/1(u)
  Downsample30/1 -> FIR Filter 25/1(u)
  Downsample31/1 -> FIR Filter 26/1(u)
  Downsample18/1 -> FIR Filter 27/1(u)
  Downsample19/1 -> FIR Filter 28/1(u)
  Downsample20/1 -> FIR Filter 29/1(u)
  Downsample21/1 -> FIR Filter 30/1(u)
  Downsample22/1 -> FIR Filter 31/1(u)
  Downsample23/1 -> FIR Filter 32/1(u)
  FIR Filter 11/1(x) -> FFT/11(In11)
  FIR Filter 12/1(x) -> FFT/12(In12)
  FIR Filter 13/1(x) -> FFT/13(In13)
  FIR Filter 14/1(x) -> FFT/14(In14)
  FIR Filter 15/1(x) -> FFT/15(In15)
  FIR Filter 16/1(x) -> FFT/16(In16)
  FIR Filter 17/1(x) -> FFT/17(In17)
  FIR Filter 18/1(x) -> FFT/18(In18)
  FIR Filter 19/1(x) -> FFT/19(In19)
  FIR Filter 20/1(x) -> FFT/20(In20)
  FIR Filter 21/1(x) -> FFT/21(In21)
  FIR Filter 22/1(x) -> FFT/22(In22)
  FIR Filter 23/1(x) -> FFT/23(In23)
  FIR Filter 24/1(x) -> FFT/24(In24)
  FIR Filter 25/1(x) -> FFT/25(In25)
  FIR Filter 26/1(x) -> FFT/26(In26)
  FIR Filter 27/1(x) -> FFT/27(In27)
  FIR Filter 28/1(x) -> FFT/28(In28)
  FIR Filter 29/1(x) -> FFT/29(In29)
  FIR Filter 30/1(x) -> FFT/30(In30)
  FIR Filter 31/1(x) -> FFT/31(In31)
  FIR Filter 32/1(x) -> FFT/32(In32)
  FFT/27(Out27) -> " CORDIC Complex to Magnitude Angle26"/1(Z)
  FFT/28(Out28) -> " CORDIC Complex to Magnitude Angle27"/1(Z)
  FFT/29(Out29) -> " CORDIC Complex to Magnitude Angle28"/1(Z)

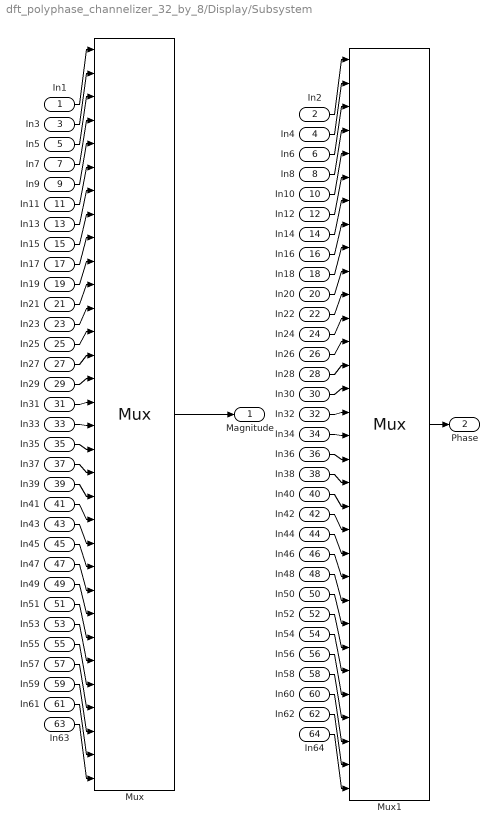
== system dft_polyphase_channelizer_32_by_8/Display/Subsystem ==
  In1 : Inport
  In2 : Inport  Port=2
  In3 : Inport  Port=3
  In4 : Inport  Port=4
  In5 : Inport  Port=5
  In6 : Inport  Port=6
  In7 : Inport  Port=7
  In8 : Inport  Port=8
  In9 : Inport  Port=9
  In10 : Inport  Port=10
  In11 : Inport  Port=11
  In12 : Inport  Port=12
  In13 : Inport  Port=13
  In14 : Inport  Port=14
  In15 : Inport  Port=15
  In16 : Inport  Port=16
  In17 : Inport  Port=17
  In18 : Inport  Port=18
  In19 : Inport  Port=19
  In20 : Inport  Port=20
  In21 : Inport  Port=21
  In22 : Inport  Port=22
  In23 : Inport  Port=23
  In24 : Inport  Port=24
  In25 : Inport  Port=25
  In26 : Inport  Port=26
  In27 : Inport  Port=27
  In28 : Inport  Port=28
  In29 : Inport  Port=29
  In30 : Inport  Port=30
  In31 : Inport  Port=31
  In32 : Inport  Port=32
  In33 : Inport  Port=33
  In34 : Inport  Port=34
  In35 : Inport  Port=35
  In36 : Inport  Port=36
  In37 : Inport  Port=37
  In38 : Inport  Port=38
  In39 : Inport  Port=39
  In40 : Inport  Port=40
  In41 : Inport  Port=41
  In42 : Inport  Port=42
  In43 : Inport  Port=43
  In44 : Inport  Port=44
  In45 : Inport  Port=45
  In46 : Inport  Port=46
  In47 : Inport  Port=47
  In48 : Inport  Port=48
  In49 : Inport  Port=49
  In50 : Inport  Port=50
  In51 : Inport  Port=51
  In52 : Inport  Port=52
  In53 : Inport  Port=53
  In54 : Inport  Port=54
  In55 : Inport  Port=55
  In56 : Inport  Port=56
  In57 : Inport  Port=57
  In58 : Inport  Port=58
  In59 : Inport  Port=59
  In60 : Inport  Port=60
  In61 : Inport  Port=61
  In62 : Inport  Port=62
  In63 : Inport  Port=63
  In64 : Inport  Port=64
  Mux : Mux  Inputs=32
  Mux1 : Mux  Inputs=32
  Magnitude : Outport
  Phase : Outport  Port=2
  wires:
  In5/1 -> Mux/3
  In2/1 -> Mux1/1
  In10/1 -> Mux1/5
  In4/1 -> Mux1/2
  In14/1 -> Mux1/7
  In12/1 -> Mux1/6
  In6/1 -> Mux1/3
  In26/1 -> Mux1/13
  In18/1 -> Mux1/9
  In46/1 -> Mux1/23
  In16/1 -> Mux1/8
  In20/1 -> Mux1/10
  In37/1 -> Mux/19
  In52/1 -> Mux1/26
  In22/1 -> Mux1/11
  In64/1 -> Mux1/32
  In42/1 -> Mux1/21
  In28/1 -> Mux1/14
  In36/1 -> Mux1/18
  In38/1 -> Mux1/19
  In40/1 -> Mux1/20
  In17/1 -> Mux/9
  In53/1 -> Mux/27
  In43/1 -> Mux/22
  In27/1 -> Mux/14
  In44/1 -> Mux1/22
  In50/1 -> Mux1/25
  In48/1 -> Mux1/24
  In55/1 -> Mux/28
  Mux1/1 -> Phase/1
  In23/1 -> Mux/12
  In54/1 -> Mux1/27
  In7/1 -> Mux/4
  In51/1 -> Mux/26
  In15/1 -> Mux/8
  In1/1 -> Mux/1
  In61/1 -> Mux/31
  In25/1 -> Mux/13
  In63/1 -> Mux/32
  In57/1 -> Mux/29
  In35/1 -> Mux/18
  In31/1 -> Mux/16
  In3/1 -> Mux/2
  In29/1 -> Mux/15
  In59/1 -> Mux/30
  In24/1 -> Mux1/12
  In13/1 -> Mux/7
  In19/1 -> Mux/10
  In9/1 -> Mux/5
  In47/1 -> Mux/24
  In56/1 -> Mux1/28
  In60/1 -> Mux1/30
  In33/1 -> Mux/17
  In39/1 -> Mux/20
  In41/1 -> Mux/21
  Mux/1 -> Magnitude/1
  In32/1 -> Mux1/16
  In8/1 -> Mux1/4
  In30/1 -> Mux1/15
  In34/1 -> Mux1/17
  In11/1 -> Mux/6
  In49/1 -> Mux/25
  In45/1 -> Mux/23
  In21/1 -> Mux/11
  In58/1 -> Mux1/29
  In62/1 -> Mux1/31

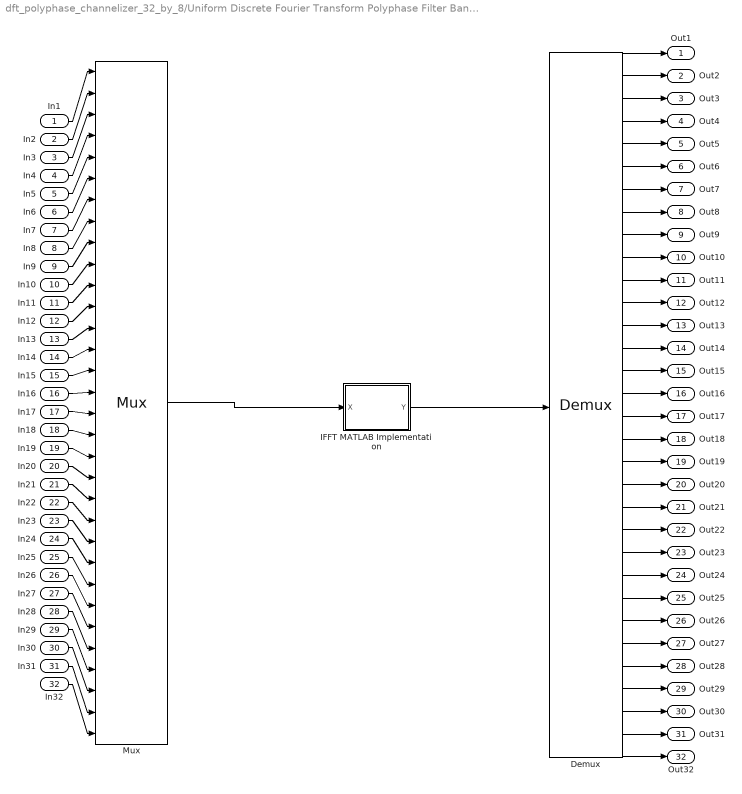
== system dft_polyphase_channelizer_32_by_8/Uniform Discrete Fourier Transform Polyphase Filter Bank/FFT ==
  In1 : Inport
  In2 : Inport  Port=2
  In3 : Inport  Port=3
  In4 : Inport  Port=4
  In5 : Inport  Port=5
  In6 : Inport  Port=6
  In7 : Inport  Port=7
  In8 : Inport  Port=8
  In9 : Inport  Port=9
  In10 : Inport  Port=10
  In11 : Inport  Port=11
  In12 : Inport  Port=12
  In13 : Inport  Port=13
  In14 : Inport  Port=14
  In15 : Inport  Port=15
  In16 : Inport  Port=16
  In17 : Inport  Port=17
  In18 : Inport  Port=18
  In19 : Inport  Port=19
  In20 : Inport  Port=20
  In21 : Inport  Port=21
  In22 : Inport  Port=22
  In23 : Inport  Port=23
  In24 : Inport  Port=24
  In25 : Inport  Port=25
  In26 : Inport  Port=26
  In27 : Inport  Port=27
  In28 : Inport  Port=28
  In29 : Inport  Port=29
  In30 : Inport  Port=30
  In31 : Inport  Port=31
  In32 : Inport  Port=32
  Demux : Demux  Outputs=32
  IFFT MATLAB Implementation : MATLAB Function  TreatAsAtomicUnit=on  mask{T=T.fft}
      mask prompts: T "Types table"
  Mux : Mux  Inputs=32
  Out1 : Outport
  Out2 : Outport  Port=2
  Out3 : Outport  Port=3
  Out4 : Outport  Port=4
  Out5 : Outport  Port=5
  Out6 : Outport  Port=6
  Out7 : Outport  Port=7
  Out8 : Outport  Port=8
  Out9 : Outport  Port=9
  Out10 : Outport  Port=10
  Out11 : Outport  Port=11
  Out12 : Outport  Port=12
  Out13 : Outport  Port=13
  Out14 : Outport  Port=14
  Out15 : Outport  Port=15
  Out16 : Outport  Port=16
  Out17 : Outport  Port=17
  Out18 : Outport  Port=18
  Out19 : Outport  Port=19
  Out20 : Outport  Port=20
  Out21 : Outport  Port=21
  Out22 : Outport  Port=22
  Out23 : Outport  Port=23
  Out24 : Outport  Port=24
  Out25 : Outport  Port=25
  Out26 : Outport  Port=26
  Out27 : Outport  Port=27
  Out28 : Outport  Port=28
  Out29 : Outport  Port=29
  Out30 : Outport  Port=30
  Out31 : Outport  Port=31
  Out32 : Outport  Port=32
  wires:
  In1/1 -> Mux/1
  In4/1 -> Mux/4
  In3/1 -> Mux/3
  In2/1 -> Mux/2
  Mux/1 -> IFFT MATLAB Implementation/1(X)
  IFFT MATLAB Implementation/1(Y) -> Demux/1
  In9/1 -> Mux/9
  In12/1 -> Mux/12
  In11/1 -> Mux/11
  In10/1 -> Mux/10
  In17/1 -> Mux/17
  In20/1 -> Mux/20
  In19/1 -> Mux/19
  In18/1 -> Mux/18
  In25/1 -> Mux/25
  In28/1 -> Mux/28
  In27/1 -> Mux/27
  In26/1 -> Mux/26
  In5/1 -> Mux/5
  In6/1 -> Mux/6
  In7/1 -> Mux/7
  In8/1 -> Mux/8
  In13/1 -> Mux/13
  In14/1 -> Mux/14
  In15/1 -> Mux/15
  In16/1 -> Mux/16
  In21/1 -> Mux/21
  In22/1 -> Mux/22
  In23/1 -> Mux/23
  In24/1 -> Mux/24
  In29/1 -> Mux/29
  In30/1 -> Mux/30
  In31/1 -> Mux/31
  In32/1 -> Mux/32
  Demux/1 -> Out1/1
  Demux/2 -> Out2/1
  Demux/3 -> Out3/1
  Demux/4 -> Out4/1
  Demux/5 -> Out5/1
  Demux/6 -> Out6/1
  Demux/7 -> Out7/1
  Demux/8 -> Out8/1
  Demux/9 -> Out9/1
  Demux/10 -> Out10/1
  Demux/11 -> Out11/1
  Demux/12 -> Out12/1
  Demux/13 -> Out13/1
  Demux/14 -> Out14/1
  Demux/15 -> Out15/1
  Demux/16 -> Out16/1
  Demux/17 -> Out17/1
  Demux/18 -> Out18/1
  Demux/19 -> Out19/1
  Demux/20 -> Out20/1
  Demux/21 -> Out21/1
  Demux/22 -> Out22/1
  Demux/23 -> Out23/1
  Demux/24 -> Out24/1
  Demux/25 -> Out25/1
  Demux/26 -> Out26/1
  Demux/27 -> Out27/1
  Demux/28 -> Out28/1
  Demux/29 -> Out29/1
  Demux/30 -> Out30/1
  Demux/31 -> Out31/1
  Demux/32 -> Out32/1

== matlab function dft_polyphase_channelizer_32_by_8/Uniform Discrete Fourier Transform Polyphase Filter Bank/ CORDIC Complex to Magnitude Angle1 ==
  data: Z input; magnitudeZ output; angleZ output
function [magnitudeZ, angleZ] = cordic_magnitude_angle(Z)
    [magnitudeZ, angleZ] = cordic_cart2pol(Z);
end

== matlab function dft_polyphase_channelizer_32_by_8/Uniform Discrete Fourier Transform Polyphase Filter Bank/ CORDIC Complex to Magnitude Angle ==
  data: Z input; magnitudeZ output; angleZ output
function [magnitudeZ, angleZ] = cordic_magnitude_angle(Z)
    [magnitudeZ, angleZ] = cordic_cart2pol(Z);
end

== matlab function dft_polyphase_channelizer_32_by_8/Uniform Discrete Fourier Transform Polyphase Filter Bank/ CORDIC Complex to Magnitude Angle10 ==
  data: Z input; magnitudeZ output; angleZ output
function [magnitudeZ, angleZ] = cordic_magnitude_angle(Z)
    [magnitudeZ, angleZ] = cordic_cart2pol(Z);
end

== matlab function dft_polyphase_channelizer_32_by_8/Uniform Discrete Fourier Transform Polyphase Filter Bank/ CORDIC Complex to Magnitude Angle11 ==
  data: Z input; magnitudeZ output; angleZ output
function [magnitudeZ, angleZ] = cordic_magnitude_angle(Z)
    [magnitudeZ, angleZ] = cordic_cart2pol(Z);
end

== matlab function dft_polyphase_channelizer_32_by_8/Uniform Discrete Fourier Transform Polyphase Filter Bank/ CORDIC Complex to Magnitude Angle12 ==
  data: Z input; magnitudeZ output; angleZ output
function [magnitudeZ, angleZ] = cordic_magnitude_angle(Z)
    [magnitudeZ, angleZ] = cordic_cart2pol(Z);
end

== matlab function dft_polyphase_channelizer_32_by_8/Uniform Discrete Fourier Transform Polyphase Filter Bank/ CORDIC Complex to Magnitude Angle13 ==
  data: Z input; magnitudeZ output; angleZ output
function [magnitudeZ, angleZ] = cordic_magnitude_angle(Z)
    [magnitudeZ, angleZ] = cordic_cart2pol(Z);
end

== matlab function dft_polyphase_channelizer_32_by_8/Uniform Discrete Fourier Transform Polyphase Filter Bank/ CORDIC Complex to Magnitude Angle14 ==
  data: Z input; magnitudeZ output; angleZ output
function [magnitudeZ, angleZ] = cordic_magnitude_angle(Z)
    [magnitudeZ, angleZ] = cordic_cart2pol(Z);
end

== matlab function dft_polyphase_channelizer_32_by_8/Uniform Discrete Fourier Transform Polyphase Filter Bank/ CORDIC Complex to Magnitude Angle15 ==
  data: Z input; magnitudeZ output; angleZ output
function [magnitudeZ, angleZ] = cordic_magnitude_angle(Z)
    [magnitudeZ, angleZ] = cordic_cart2pol(Z);
end

== matlab function dft_polyphase_channelizer_32_by_8/Uniform Discrete Fourier Transform Polyphase Filter Bank/ CORDIC Complex to Magnitude Angle16 ==
  data: Z input; magnitudeZ output; angleZ output
function [magnitudeZ, angleZ] = cordic_magnitude_angle(Z)
    [magnitudeZ, angleZ] = cordic_cart2pol(Z);
end

== matlab function dft_polyphase_channelizer_32_by_8/Uniform Discrete Fourier Transform Polyphase Filter Bank/ CORDIC Complex to Magnitude Angle17 ==
  data: Z input; magnitudeZ output; angleZ output
function [magnitudeZ, angleZ] = cordic_magnitude_angle(Z)
    [magnitudeZ, angleZ] = cordic_cart2pol(Z);
end

== matlab function dft_polyphase_channelizer_32_by_8/Uniform Discrete Fourier Transform Polyphase Filter Bank/ CORDIC Complex to Magnitude Angle18 ==
  data: Z input; magnitudeZ output; angleZ output
function [magnitudeZ, angleZ] = cordic_magnitude_angle(Z)
    [magnitudeZ, angleZ] = cordic_cart2pol(Z);
end

== matlab function dft_polyphase_channelizer_32_by_8/Uniform Discrete Fourier Transform Polyphase Filter Bank/ CORDIC Complex to Magnitude Angle19 ==
  data: Z input; magnitudeZ output; angleZ output
function [magnitudeZ, angleZ] = cordic_magnitude_angle(Z)
    [magnitudeZ, angleZ] = cordic_cart2pol(Z);
end

== matlab function dft_polyphase_channelizer_32_by_8/Uniform Discrete Fourier Transform Polyphase Filter Bank/ CORDIC Complex to Magnitude Angle2 ==
  data: Z input; magnitudeZ output; angleZ output
function [magnitudeZ, angleZ] = cordic_magnitude_angle(Z)
    [magnitudeZ, angleZ] = cordic_cart2pol(Z);
end

== matlab function dft_polyphase_channelizer_32_by_8/Uniform Discrete Fourier Transform Polyphase Filter Bank/ CORDIC Complex to Magnitude Angle20 ==
  data: Z input; magnitudeZ output; angleZ output
function [magnitudeZ, angleZ] = cordic_magnitude_angle(Z)
    [magnitudeZ, angleZ] = cordic_cart2pol(Z);
end

== matlab function dft_polyphase_channelizer_32_by_8/Uniform Discrete Fourier Transform Polyphase Filter Bank/ CORDIC Complex to Magnitude Angle21 ==
  data: Z input; magnitudeZ output; angleZ output
function [magnitudeZ, angleZ] = cordic_magnitude_angle(Z)
    [magnitudeZ, angleZ] = cordic_cart2pol(Z);
end

== matlab function dft_polyphase_channelizer_32_by_8/Uniform Discrete Fourier Transform Polyphase Filter Bank/ CORDIC Complex to Magnitude Angle22 ==
  data: Z input; magnitudeZ output; angleZ output
function [magnitudeZ, angleZ] = cordic_magnitude_angle(Z)
    [magnitudeZ, angleZ] = cordic_cart2pol(Z);
end

== matlab function dft_polyphase_channelizer_32_by_8/Uniform Discrete Fourier Transform Polyphase Filter Bank/ CORDIC Complex to Magnitude Angle23 ==
  data: Z input; magnitudeZ output; angleZ output
function [magnitudeZ, angleZ] = cordic_magnitude_angle(Z)
    [magnitudeZ, angleZ] = cordic_cart2pol(Z);
end

== matlab function dft_polyphase_channelizer_32_by_8/Uniform Discrete Fourier Transform Polyphase Filter Bank/ CORDIC Complex to Magnitude Angle24 ==
  data: Z input; magnitudeZ output; angleZ output
function [magnitudeZ, angleZ] = cordic_magnitude_angle(Z)
    [magnitudeZ, angleZ] = cordic_cart2pol(Z);
end

== matlab function dft_polyphase_channelizer_32_by_8/Uniform Discrete Fourier Transform Polyphase Filter Bank/ CORDIC Complex to Magnitude Angle25 ==
  data: Z input; magnitudeZ output; angleZ output
function [magnitudeZ, angleZ] = cordic_magnitude_angle(Z)
    [magnitudeZ, angleZ] = cordic_cart2pol(Z);
end

== matlab function dft_polyphase_channelizer_32_by_8/Uniform Discrete Fourier Transform Polyphase Filter Bank/ CORDIC Complex to Magnitude Angle26 ==
  data: Z input; magnitudeZ output; angleZ output
function [magnitudeZ, angleZ] = cordic_magnitude_angle(Z)
    [magnitudeZ, angleZ] = cordic_cart2pol(Z);
end

== matlab function dft_polyphase_channelizer_32_by_8/Uniform Discrete Fourier Transform Polyphase Filter Bank/ CORDIC Complex to Magnitude Angle27 ==
  data: Z input; magnitudeZ output; angleZ output
function [magnitudeZ, angleZ] = cordic_magnitude_angle(Z)
    [magnitudeZ, angleZ] = cordic_cart2pol(Z);
end

== matlab function dft_polyphase_channelizer_32_by_8/Uniform Discrete Fourier Transform Polyphase Filter Bank/ CORDIC Complex to Magnitude Angle28 ==
  data: Z input; magnitudeZ output; angleZ output
function [magnitudeZ, angleZ] = cordic_magnitude_angle(Z)
    [magnitudeZ, angleZ] = cordic_cart2pol(Z);
end

== matlab function dft_polyphase_channelizer_32_by_8/Uniform Discrete Fourier Transform Polyphase Filter Bank/ CORDIC Complex to Magnitude Angle29 ==
  data: Z input; magnitudeZ output; angleZ output
function [magnitudeZ, angleZ] = cordic_magnitude_angle(Z)
    [magnitudeZ, angleZ] = cordic_cart2pol(Z);
end

== matlab function dft_polyphase_channelizer_32_by_8/Uniform Discrete Fourier Transform Polyphase Filter Bank/ CORDIC Complex to Magnitude Angle3 ==
  data: Z input; magnitudeZ output; angleZ output
function [magnitudeZ, angleZ] = cordic_magnitude_angle(Z)
    [magnitudeZ, angleZ] = cordic_cart2pol(Z);
end

== matlab function dft_polyphase_channelizer_32_by_8/Uniform Discrete Fourier Transform Polyphase Filter Bank/ CORDIC Complex to Magnitude Angle30 ==
  data: Z input; magnitudeZ output; angleZ output
function [magnitudeZ, angleZ] = cordic_magnitude_angle(Z)
    [magnitudeZ, angleZ] = cordic_cart2pol(Z);
end

== matlab function dft_polyphase_channelizer_32_by_8/Uniform Discrete Fourier Transform Polyphase Filter Bank/ CORDIC Complex to Magnitude Angle31 ==
  data: Z input; magnitudeZ output; angleZ output
function [magnitudeZ, angleZ] = cordic_magnitude_angle(Z)
    [magnitudeZ, angleZ] = cordic_cart2pol(Z);
end

== matlab function dft_polyphase_channelizer_32_by_8/Uniform Discrete Fourier Transform Polyphase Filter Bank/ CORDIC Complex to Magnitude Angle4 ==
  data: Z input; magnitudeZ output; angleZ output
function [magnitudeZ, angleZ] = cordic_magnitude_angle(Z)
    [magnitudeZ, angleZ] = cordic_cart2pol(Z);
end

== matlab function dft_polyphase_channelizer_32_by_8/Uniform Discrete Fourier Transform Polyphase Filter Bank/ CORDIC Complex to Magnitude Angle5 ==
  data: Z input; magnitudeZ output; angleZ output
function [magnitudeZ, angleZ] = cordic_magnitude_angle(Z)
    [magnitudeZ, angleZ] = cordic_cart2pol(Z);
end

== matlab function dft_polyphase_channelizer_32_by_8/Uniform Discrete Fourier Transform Polyphase Filter Bank/ CORDIC Complex to Magnitude Angle6 ==
  data: Z input; magnitudeZ output; angleZ output
function [magnitudeZ, angleZ] = cordic_magnitude_angle(Z)
    [magnitudeZ, angleZ] = cordic_cart2pol(Z);
end

== matlab function dft_polyphase_channelizer_32_by_8/Uniform Discrete Fourier Transform Polyphase Filter Bank/ CORDIC Complex to Magnitude Angle7 ==
  data: Z input; magnitudeZ output; angleZ output
function [magnitudeZ, angleZ] = cordic_magnitude_angle(Z)
    [magnitudeZ, angleZ] = cordic_cart2pol(Z);
end
